simulink model "AFS_Master_Runner"  (R2020b)
settings: configuration reference "VLS_Standard_Configuration" (kept outside this file)
settings Model: DataDictionary=AFS_Master_Model.sldd  Creator=mmoufakk  LastModifiedBy=smettupa
settings ConfigSetRef: SourceName=VLS_Standard_Configuration

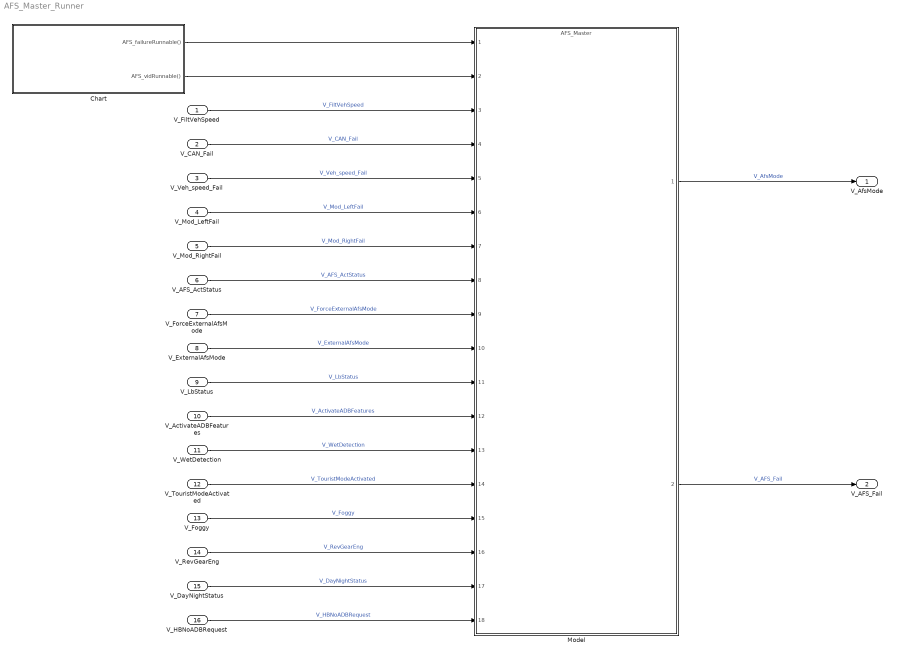
== system AFS_Master_Runner ==
  V_FiltVehSpeed : Inport
  V_CAN_Fail : Inport  Port=2
  V_Veh_speed_Fail : Inport  Port=3
  V_Mod_LeftFail : Inport  Port=4
  V_Mod_RightFail : Inport  Port=5
  V_AFS_ActStatus : Inport  Port=6
  V_ForceExternalAfsMode : Inport  Port=7
  V_ExternalAfsMode : Inport  Port=8
  V_LbStatus : Inport  Port=9
  V_ActivateADBFeatures : Inport  Port=10
  V_WetDetection : Inport  Port=11
  V_TouristModeActivated : Inport  Port=12
  V_Foggy : Inport  Port=13
  V_RevGearEng : Inport  Port=14
  V_DayNightStatus : Inport  Port=15
  V_HBNoADBRequest : Inport  Port=16
  Chart : Stateflow chart  TreatAsAtomicUnit=on
  Model : ModelReference  ModelNameDialog=AFS_Master.slx  SimulationMode=Normal  ScheduleRates=on  ModelReferenceVersion=1.129
  V_AfsMode : Outport  PortDimensions=1
  V_AFS_Fail : Outport  Port=2  VectorParamsAs1DForOutWhenUnconnected=off
  wires:
  Chart/2(AFS_vidRunnable()) -> Model/2
  Chart/1(AFS_failureRunnable()) -> Model/1
  V_FiltVehSpeed/1 -> Model/3  "V_FiltVehSpeed"
  V_CAN_Fail/1 -> Model/4  "V_CAN_Fail"
  V_Veh_speed_Fail/1 -> Model/5  "V_Veh_speed_Fail"
  V_AFS_ActStatus/1 -> Model/8  "V_AFS_ActStatus"
  V_LbStatus/1 -> Model/11  "V_LbStatus"
  V_ActivateADBFeatures/1 -> Model/12  "V_ActivateADBFeatures"
  V_WetDetection/1 -> Model/13  "V_WetDetection"
  V_TouristModeActivated/1 -> Model/14  "V_TouristModeActivated"
  V_Foggy/1 -> Model/15  "V_Foggy"
  V_RevGearEng/1 -> Model/16  "V_RevGearEng"
  V_DayNightStatus/1 -> Model/17  "V_DayNightStatus"
  V_HBNoADBRequest/1 -> Model/18  "V_HBNoADBRequest"
  Model/1 -> V_AfsMode/1  "V_AfsMode"
  V_ForceExternalAfsMode/1 -> Model/9  "V_ForceExternalAfsMode"
  Model/2 -> V_AFS_Fail/1  "V_AFS_Fail"
  V_Mod_LeftFail/1 -> Model/6  "V_Mod_LeftFail"
  V_Mod_RightFail/1 -> Model/7  "V_Mod_RightFail"
  V_ExternalAfsMode/1 -> Model/10  "V_ExternalAfsMode"

== stateflow chart AFS_Master_Runner/Chart ==
  state Scheduler
    on every(1,tick):
    send(AFS_failureRunnable);
    on every(2,tick):
    send(AFS_vidRunnable);
  (default) -> Scheduler
  events: AFS_failureRunnable output FUNCTION_CALL_EVENT; AFS_vidRunnable output FUNCTION_CALL_EVENT
